simulink model "sin"  (R2016b)
settings: Solver=VariableStepAuto  StartTime=0.0  StopTime=10.0  RelTol=1e-3
settings Model: Creator=96919  LastModifiedBy=96919

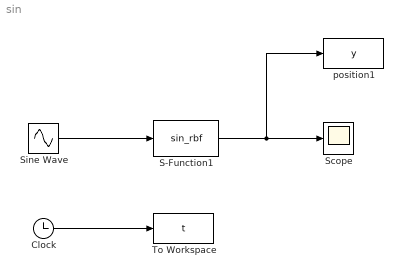
== system sin ==
  Clock : Clock
  S-Function1 : S-Function  FunctionName=sin_rbf  SFunctionDeploymentMode=off  EnableBusSupport=off
  Scope : Scope
  Sine Wave : Sin  SampleTime=0
  To Workspace : ToWorkspace  VariableName=t  SampleTime=-1
  position1 : ToWorkspace  VariableName=y  SampleTime=-1
  wires:
  Sine Wave/1 -> S-Function1/1
  S-Function1/1 -> position1/1, Scope/1
  Clock/1 -> To Workspace/1
